simulink model "Switchig_verificatio"  (R2015a)
settings: Solver=ode45  StartTime=0.0  StopTime=1.0  MaxStep=0.0000001  MinStep=0.00000001  RelTol=1e-3
libraries: simulink x1, powerlib x1
settings Model: Creator=hp  LastModifiedBy=hp

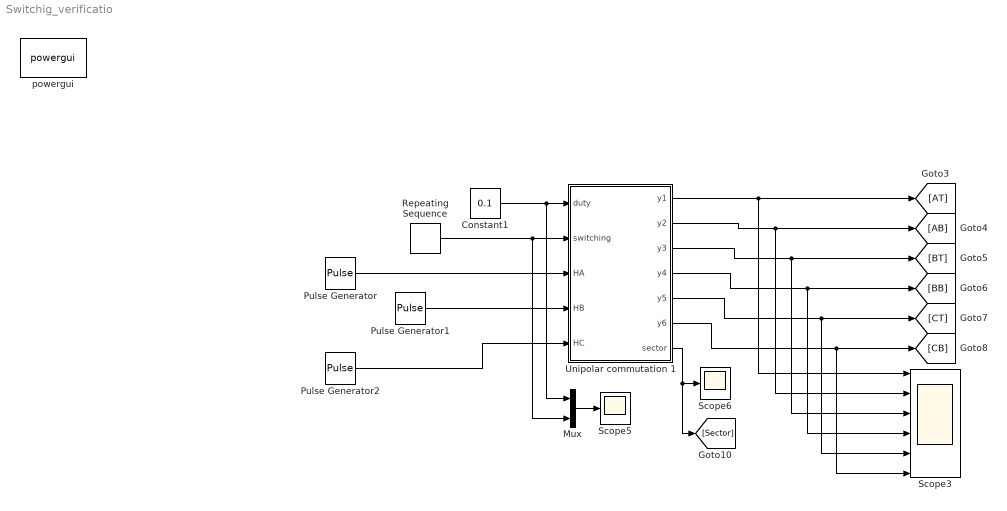
== system Switchig_verificatio ==
  Constant1 : Constant  Value=0.1
  Mux : Mux  Inputs=2
  Pulse Generator : DiscretePulseGenerator  PulseType=Time based  Period=0.1  PulseWidth=50
  Pulse Generator1 : DiscretePulseGenerator  PulseType=Time based  Period=0.1  PulseWidth=50  PhaseDelay=0.1/3
  Pulse Generator2 : DiscretePulseGenerator  PulseType=Time based  Period=0.1  PulseWidth=50  PhaseDelay=0.2/3
  Repeating Sequence : simulink/Sources/Repeating Sequence  rep_seq_t=[0 1]/10000  rep_seq_y=[0 1]
  Scope3 : Scope  NumInputPorts=6
      settings: YMin=-1~0.95~-1~-1~0.95~-1  YMax=1~1.05~1~1~1.05~1  SaveName=ScopeData3
  Scope5 : Scope
      settings: YMin=2.77556e-17  YMax=1  SaveName=ScopeData5
  Scope6 : Scope
      settings: YMin=3.8  YMax=4.2  SaveName=ScopeData6
  Unipolar commutation 1 : MATLAB Function  TreatAsAtomicUnit=on
  powergui : powerlib/powergui  Priority=1  SimulationMode=Discrete  SolverType=Tustin/Backward Euler (TBE)  SampleTime=1e-6  frequency=60  SPID=off  DisableSnubberDevices=off  DisableRonSwitches=off  DisableVfSwitches=off  SwTol=0  DisplayEquations=off  Interpol=off  methode=off  Ts=100  FunctionMessages=off  echomessages=off  HookPort=off  EnableUseOfTLC=off  x0status=blocks  frequencyindice=0  Pbase=100e6  ErrMax=1e-4  Iterations=50  UnitsV=kV  UnitsW=MW  buscounter=0  RestoreLinks=warning  ResistiveCurrentMeasurement=off  Frange=[0:2:500]  Ylog=off  Xlog=on  ShowGrid=off  save=off  variable=ZData  structure=0  ZoomFFT=off  StartTime=0.0  cycles=1  DisplayStyle=1  fundamental=60  FreqAxis=off  MaxFrequency=1000  frequencyindicesteady=1  RmsSteady=1  display=off
  wires:
  Repeating Sequence/1 -> Unipolar commutation 1/2(switching), Mux/2
  Unipolar commutation 1/1(y1) -> Scope3/1, [AT]
  Unipolar commutation 1/2(y2) -> Scope3/2, [AB]
  Unipolar commutation 1/3(y3) -> Scope3/3, [BT]
  Unipolar commutation 1/4(y4) -> Scope3/4, [BB]
  Unipolar commutation 1/5(y5) -> Scope3/5, [CT]
  Unipolar commutation 1/6(y6) -> Scope3/6, [CB]
  Mux/1 -> Scope5/1
  Unipolar commutation 1/7(sector) -> [Sector], Scope6/1
  Constant1/1 -> Unipolar commutation 1/1(duty), Mux/1
  Pulse Generator/1 -> Unipolar commutation 1/3(HA)
  Pulse Generator1/1 -> Unipolar commutation 1/4(HB)
  Pulse Generator2/1 -> Unipolar commutation 1/5(HC)

== matlab function Switchig_verificatio/Unipolar commutation 1 ==
  data: duty input; y1 output; switching input; HA input; HB input; HC input; y2 output; y3 output; y4 output; y5 output; y6 output; sector output
function [y1,y2,y3,y4,y5,y6,sector] = fcn(duty,switching, HA,HB,HC)
%#codegen
hall_state = (HA*4)+(HB*2)+(HC);
if hall_state==4                %sector 1
    if duty>switching           %V +ve W -ve
        y3 = 1;
        y1 = 0;
        y2 = 0;
        y4 = 0;
        y5 = 0;
    else
        y4 = 1;
        y1 = 0;
        y2 = 0;
        y3 = 0;
        y5 = 0;
    end
    y6 = 1;
    
elseif hall_state==6                %sector 2
    if duty>switching           %V +ve u -ve 
        y3 = 1;
        y1 = 0;
        y5 = 0;
        y6 = 0;
        y4 = 0;
    else
        y4 = 1;
        y1 = 0;
        y5 = 0;
        y6 = 0;
        y3 = 0;
    end
    y2 = 1;
elseif hall_state==2                %sector 3
    if duty>switching             %W +ve U -ve
        y5 = 1;
        y1 = 0;
        y3 = 0;
        y4 = 0;
        y6 = 0;
    else
        y6 = 1;
        y1 = 0;
        y3 = 0;
        y4 = 0;
        y5 = 0;
    end
    y2 = 1;
elseif hall_state==3                %sector 4
    if duty>switching           %W +ve V -ve
        y5 = 1;
        y1 = 0;
        y2 = 0;
        y3 = 0;
        y6 = 0;
    else
        y6 = 1;
        y1 = 0;
        y2 = 0;
        y3 = 0;
        y5 = 0;
    end
    y4 = 1;
elseif hall_state==1                %sector 5
    if duty>switching            %U +ve V -ve
        y1 = 1;
        y2 = 0;
        y3 = 0;
        y5 = 0;
        y6 = 0;
    else
        y2 = 1;
        y1 = 0;
        y3 = 0;
        y5 = 0;
        y6 = 0;
    end
    y4 = 1;
elseif hall_state==5                %sector 6
    if duty>switching             %U +ve W -ve
        y1 = 1;
        y2 = 0;
        y3 = 0;
        y4 = 0;
        y5 = 0;
    else
        y2 = 1;
        y1 = 0;
        y3 = 0;
        y4 = 0;
        y5 = 0;
    end
    y6 = 1;
else 
        y1 = 0;
        y2 = 0;
        y3 = 0;
        y4 = 0;
        y5 = 0;
        y6 = 0;
end    
sector = hall_state;
end
